simulink model "lab4"  (R2021b)
settings: Solver=ode45  StartTime=0.0  StopTime=500  RelTol=1e-3  EnableMultiTasking=on
settings Model: Creator=user  LastModifiedBy=Lapte
settings SolverCC: AlgebraicLoopSolver=TrustRegion
settings DataIOCC: LimitDataPoints=on  SaveFormat=Array  ReturnWorkspaceOutputs=off
settings OptimizationCC: LifeSpan=inf
settings DebuggingCC: SolverPrmCheckMsg=warning  SFUnexpectedBacktrackingDiag=warning  SFNoUnconditionalDefaultTransitionDiag=warning  SFExecutionAtInitializationDiag=none  SFMachineParentedDataDiag=warning  ArithmeticOperatorsInVariantConditions=warning
settings HardwareCC: ProdBitPerPointer=32  ProdBitPerSizeT=32  ProdBitPerPtrDiffT=32  ProdLargestAtomicFloat=None  ProdIntDivRoundTo=Undefined  ProdEndianess=Unspecified  ProdWordSize=32  ProdHWDeviceType=32-bit Generic
settings ModelReferenceCC: PropagateSignalLabelsOutOfModel=off
settings SFSimCC: SimUseLocalCustomCode=off  CustomCodeUndefinedFunction=UseInterfaceOnly
settings RTWCC: RTWUseLocalCustomCode=off
settings CodeAppCC: StateflowObjectComments=on
settings GRTTargetCC: TargetLangStandard=C89/C90 (ANSI)
settings ConfigComp: CovMetricSettings=dw  CovSaveCumulativeToWorkspaceVar=on  CovSaveSingleToWorkspaceVar=on  CovExternalEMLEnable=off  CovSFcnEnable=off

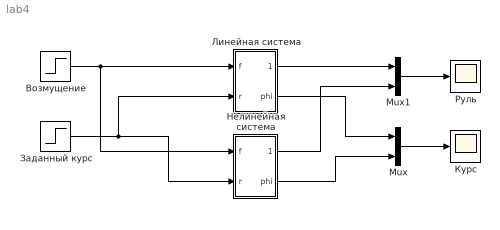
== system lab4 ==
  Mux : Mux  Inputs=2
  Mux1 : Mux  Inputs=2
  Возмущение : Step  Time=0  After=0  SampleTime=0
  Заданный курс : Step  Time=0  After=90  SampleTime=0
  Курс : Scope
  Линейная система : Subsystem
  Нелинейная система : Subsystem
  Руль : Scope
  wires:
  Возмущение/1 -> Нелинейная система/1(f), Линейная система/1(f)
  Заданный курс/1 -> Линейная система/2(r), Нелинейная система/2(r)
  Линейная система/1(delta) -> Mux1/1
  Линейная система/2(phi) -> Mux/1
  Нелинейная система/1(delta) -> Mux1/2
  Нелинейная система/2(phi) -> Mux/2
  Mux1/1 -> Руль/1
  Mux/1 -> Курс/1

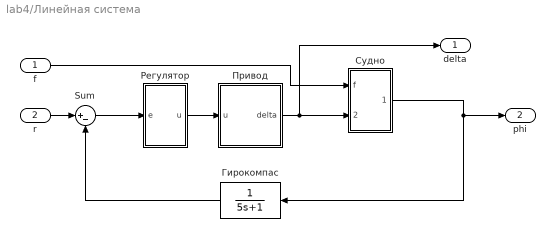
== system lab4/Линейная система ==
  f : Inport
  r : Inport  Port=2
  Sum : Sum  Inputs=|+-
  Гирокомпас : TransferFcn  Denominator=[5 1]
  Привод : Subsystem
  Регулятор : Subsystem
  Судно : Subsystem
  delta : Outport
  phi : Outport  Port=2
  wires:
  Регулятор/1(u) -> Привод/1(u)
  Судно/1(phi) -> phi/1, Гирокомпас/1
  Гирокомпас/1 -> Sum/2
  Sum/1 -> Регулятор/1(e)
  Привод/1(delta) -> delta/1, Судно/2(delta)
  r/1 -> Sum/1
  f/1 -> Судно/1(f)

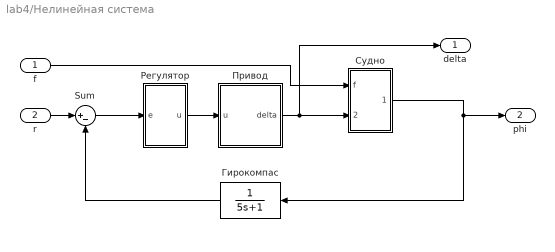
== system lab4/Нелинейная система ==
  f : Inport
  r : Inport  Port=2
  Sum : Sum  Inputs=|+-
  Гирокомпас : TransferFcn  Denominator=[5 1]
  Привод : Subsystem
  Регулятор : Subsystem
  Судно : Subsystem
  delta : Outport
  phi : Outport  Port=2
  wires:
  f/1 -> Судно/1(f)
  r/1 -> Sum/1
  Привод/1(delta) -> Судно/2(delta), delta/1
  Sum/1 -> Регулятор/1(e)
  Гирокомпас/1 -> Sum/2
  Судно/1(phi) -> Гирокомпас/1, phi/1
  Регулятор/1(u) -> Привод/1(u)

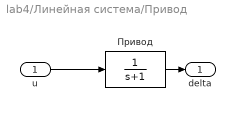
== system lab4/Линейная система/Привод ==
  u : Inport
  Привод : TransferFcn  Denominator=[1 1]
  delta : Outport
  wires:
  Привод/1 -> delta/1
  u/1 -> Привод/1

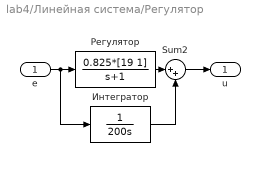
== system lab4/Линейная система/Регулятор ==
  e : Inport
  Sum2 : Sum  Inputs=|++
  Интегратор : TransferFcn  Denominator=[200 0]
  Регулятор : TransferFcn  Numerator=0.825*[19 1]  Denominator=[1 1]
  u : Outport
  wires:
  Интегратор/1 -> Sum2/2
  e/1 -> Интегратор/1, Регулятор/1
  Регулятор/1 -> Sum2/1
  Sum2/1 -> u/1

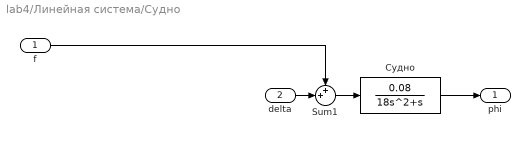
== system lab4/Линейная система/Судно ==
  f : Inport
  delta : Inport  Port=2
  Sum1 : Sum  Inputs=++|
  Судно : TransferFcn  Numerator=[0.08]  Denominator=[18 1 0]
  phi : Outport
  wires:
  delta/1 -> Sum1/2
  Sum1/1 -> Судно/1
  f/1 -> Sum1/1
  Судно/1 -> phi/1

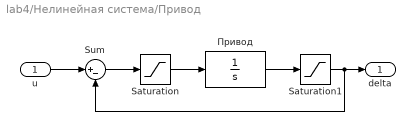
== system lab4/Нелинейная система/Привод ==
  u : Inport
  Saturation : Saturate  UpperLimit=3  LowerLimit=-3
  Saturation1 : Saturate  UpperLimit=30  LowerLimit=-30
  Sum : Sum  Inputs=|+-
  Привод : TransferFcn  Denominator=[1 0]
  delta : Outport
  wires:
  Sum/1 -> Saturation/1
  u/1 -> Sum/1
  Saturation/1 -> Привод/1
  Привод/1 -> Saturation1/1
  Saturation1/1 -> delta/1, Sum/2

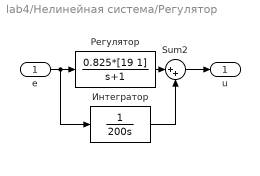
== system lab4/Нелинейная система/Регулятор ==
  e : Inport
  Sum2 : Sum  Inputs=|++
  Интегратор : TransferFcn  Denominator=[200 0]
  Регулятор : TransferFcn  Numerator=0.825*[19 1]  Denominator=[1 1]
  u : Outport
  wires:
  Sum2/1 -> u/1
  Регулятор/1 -> Sum2/1
  e/1 -> Регулятор/1, Интегратор/1
  Интегратор/1 -> Sum2/2

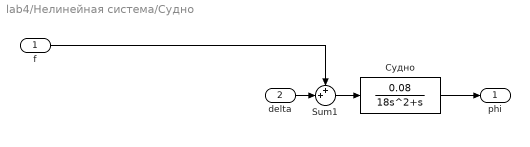
== system lab4/Нелинейная система/Судно ==
  f : Inport
  delta : Inport  Port=2
  Sum1 : Sum  Inputs=++|
  Судно : TransferFcn  Numerator=[0.08]  Denominator=[18 1 0]
  phi : Outport
  wires:
  Судно/1 -> phi/1
  f/1 -> Sum1/1
  Sum1/1 -> Судно/1
  delta/1 -> Sum1/2
